simulink model "NetworkedControlSystemBasic_Part3"  (R2023b)
settings: Solver=FixedStepAuto  StartTime=0.0  StopTime=Tsim  FixedStep=Ts  RelTol=1e-3
values from neighbouring files (symbols this model uses):
  A = [0.9719 -0.0013;-0.0340 0.8628]    [Main_Part3.m]
  B = [-0.0839 0.0232;0.0761 0.4144]    [Main_Part3.m]
  C = [0 1]    [Main_Part3.m]
  D = [0 0]    [Main_Part3.m]
  K = lqi(sys,Q_LQI,R_LQ,0)    [Main_Part3.m]
  reference_time_vec = [0 100 250]    [Main_Part3.m]
  reference_value_vec = [0 10 17]    [Main_Part3.m]
  standardDeviationMeasurementNoise = 0.04    [Main_Part3.m]
  standardDeviationProcessNoise = 0.007    [Main_Part3.m]
  Ts = 1    [Main_Part3.m]
  x0 = zeros(size(A,1),1)    [Main_Part3.m]
  x0_hat = zeros(size(A,1),1)    [Main_Part3.m]
undefined symbols (not defined in the file or in its folder): DiscIntNeverNeededParam, L
settings Model: Creator=mehra  LastModifiedBy=amior
settings SolverCC: AlgebraicLoopSolver=TrustRegion
settings DebuggingCC: UnconnectedInputMsg=warning  UnconnectedOutputMsg=warning  UnconnectedLineMsg=warning
settings ModelReferenceCC: EnableRefExpFcnMdlSchedulingChecks=on
settings RTWCC: DLArmComputeVersion=19.05

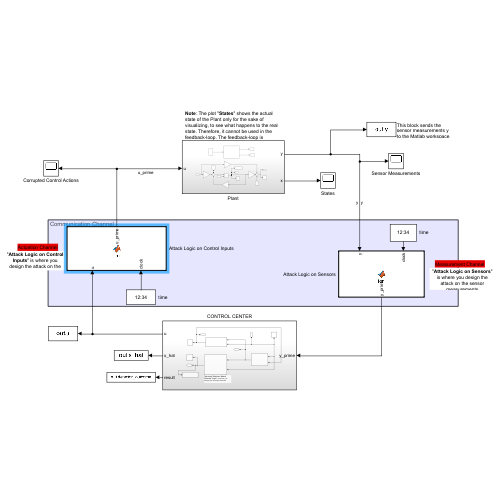
[thumbnail: Simulink's stored preview of the top-level diagram]
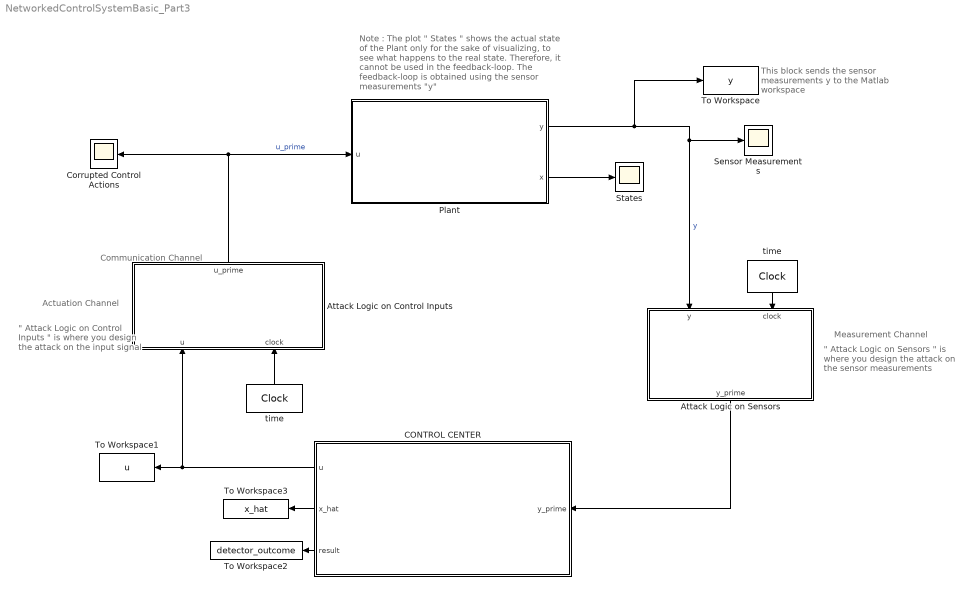
== system NetworkedControlSystemBasic_Part3 ==
  note: Note : The plot " States " shows the actual state of the Plant only for the sake of visualizing, to see what happens to the real state. Therefore, it cannot be used in the feedback-loop. The feedback-loop is obtained using the sensor measurements "y"
  note: Measurement Channel
  note: Actuation Channel
  note: Communication Channel
  note: " Attack Logic on Control Inputs " is where you design the attack on the input signal
  note: " Attack Logic on Sensors " is where you design the attack on the sensor measurements
  note: This block sends the sensor measurements y to the Matlab workspace
  Attack Logic on Control Inputs : MATLAB Function  TreatAsAtomicUnit=on
  Attack Logic on Sensors : MATLAB Function  TreatAsAtomicUnit=on
  CONTROL CENTER : Subsystem
  Corrupted Control Actions : Scope
  Plant : Subsystem
  "Sensor Measurements " : Scope
  States : Scope
  To Workspace : ToWorkspace  VariableName=y  SaveFormat=Structure With Time  SampleTime=Ts
  To Workspace1 : ToWorkspace  VariableName=u  SaveFormat=Structure With Time  SampleTime=Ts
  To Workspace2 : ToWorkspace  VariableName=detector_outcome  SaveFormat=Structure With Time  SampleTime=Ts
  To Workspace3 : ToWorkspace  VariableName=x_hat  SaveFormat=Structure With Time  SampleTime=Ts
  time : DigitalClock  SampleTime=Ts
  "time " : DigitalClock  SampleTime=Ts
  wires:
  "time "/1 -> Attack Logic on Sensors/2(clock)
  Attack Logic on Control Inputs/1(u_prime) -> Plant/1(u), Corrupted Control Actions/1  "u_prime"
  Plant/1(y) -> To Workspace/1, "Sensor Measurements "/1, Attack Logic on Sensors/1(y)  "y"
  time/1 -> Attack Logic on Control Inputs/2(clock)
  Plant/2(x) -> States/1
  CONTROL CENTER/1(u) -> Attack Logic on Control Inputs/1(u), To Workspace1/1
  Attack Logic on Sensors/1(y_prime) -> CONTROL CENTER/1(y_prime)
  CONTROL CENTER/2(x_hat) -> To Workspace3/1
  CONTROL CENTER/3(result) -> To Workspace2/1

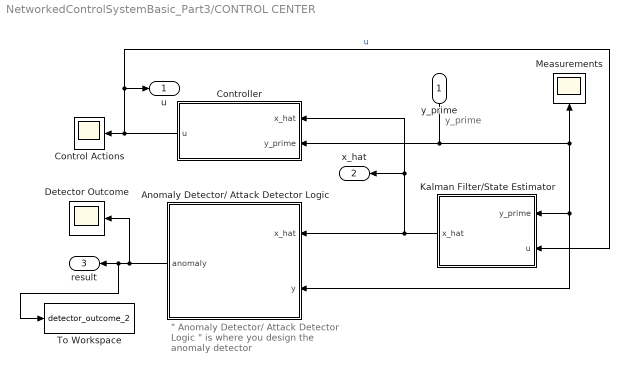
== system NetworkedControlSystemBasic_Part3/CONTROL CENTER ==
  note: y_prime
  note: " Anomaly Detector/ Attack Detector Logic " is where you design the anomaly detector
  y_prime : Inport
  Anomaly Detector/ Attack Detector Logic : MATLAB Function  TreatAsAtomicUnit=on
  Control Actions : Scope
  Controller : Subsystem
  Detector Outcome : Scope
  Kalman Filter/State Estimator : Subsystem
  Measurements : Scope
  To Workspace : ToWorkspace  VariableName=detector_outcome_2  SaveFormat=Structure With Time  SampleTime=-1
  u : Outport
  x_hat : Outport  Port=2
  result : Outport  Port=3
  wires:
  y_prime/1 -> Controller/2(y_prime), Kalman Filter/State Estimator/1(y_prime), Anomaly Detector/ Attack Detector Logic/2(y), Measurements/1
  Anomaly Detector/ Attack Detector Logic/1(anomaly) -> Detector Outcome/1, To Workspace/1, result/1
  Controller/1(u) -> u/1, Kalman Filter/State Estimator/2(u), Control Actions/1  "u"
  Kalman Filter/State Estimator/1(x_hat) -> Controller/1(x_hat), x_hat/1, Anomaly Detector/ Attack Detector Logic/1(x_hat)

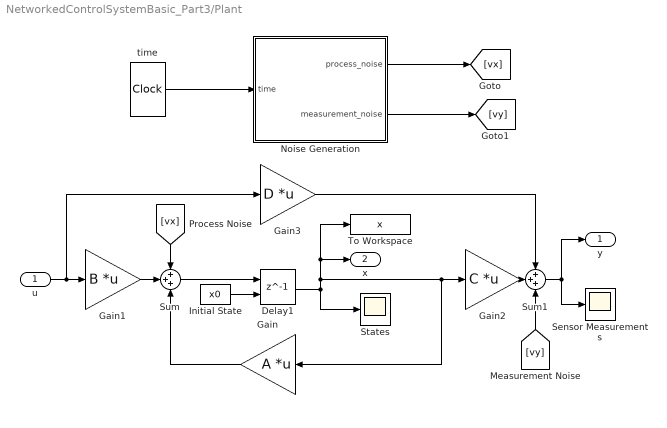
== system NetworkedControlSystemBasic_Part3/Plant ==
  u : Inport
  Delay1 : Delay  DelayLength=1  InitialConditionSource=Input port  InitialCondition=x0  SampleTime=Ts
      settings: InputPortMap=u0,p4
  Gain : Gain  Gain=A  Multiplication=Matrix(K*u)
  Gain1 : Gain  Gain=B  Multiplication=Matrix(K*u)
  Gain2 : Gain  Gain=C  Multiplication=Matrix(K*u)
  Gain3 : Gain  Gain=D  Multiplication=Matrix(K*u)
  Initial State : Constant  Value=x0
  Noise Generation : Subsystem
  Sensor Measurements : Scope
  States : Scope
  Sum : Sum  Inputs=+++
  Sum1 : Sum  Inputs=+++
  To Workspace : ToWorkspace  VariableName=x  SaveFormat=Structure With Time  SampleTime=Ts
  "time " : DigitalClock  SampleTime=Ts
  y : Outport  VectorParamsAs1DForOutWhenUnconnected=off
  x : Outport  Port=2  VectorParamsAs1DForOutWhenUnconnected=off
  wires:
  "time "/1 -> Noise Generation/1(time)
  Noise Generation/1(process_noise) -> [vx]
  Noise Generation/2(measurement_noise) -> [vy]
  Delay1/1 -> Gain2/1, Gain/1, x/1, To Workspace/1, States/1
  Sum/1 -> Delay1/1
  Gain/1 -> Sum/3
  Gain1/1 -> Sum/2
  u/1 -> Gain3/1, Gain1/1
  Gain2/1 -> Sum1/2
  Gain3/1 -> Sum1/1
  Sum1/1 -> Sensor Measurements/1, y/1
  [vx] -> Sum/1
  [vy] -> Sum1/3
  Initial State/1 -> Delay1/2

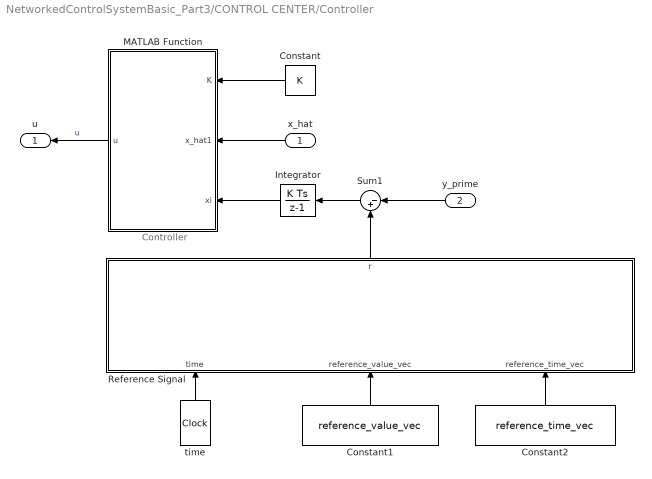
== system NetworkedControlSystemBasic_Part3/CONTROL CENTER/Controller ==
  note: Controller
  x_hat : Inport
  y_prime : Inport  Port=2
  Constant : Constant  Value=K  VectorParams1D=off
  Constant1 : Constant  Value=reference_value_vec  VectorParams1D=off
  Constant2 : Constant  Value=reference_time_vec  VectorParams1D=off
  Integrator : DiscreteIntegrator  SampleTime=Ts  ICPrevOutput=DiscIntNeverNeededParam  ICPrevScaledInput=DiscIntNeverNeededParam
  MATLAB Function : MATLAB Function  TreatAsAtomicUnit=on
  Reference Signal : MATLAB Function  TreatAsAtomicUnit=on
  Sum1 : Sum  Inputs=|-+
  "time   " : DigitalClock  SampleTime=Ts
  u : Outport  VectorParamsAs1DForOutWhenUnconnected=off
  wires:
  Sum1/1 -> Integrator/1
  x_hat/1 -> MATLAB Function/2(x_hat1)
  MATLAB Function/1(u) -> u/1  "u"
  y_prime/1 -> Sum1/1
  Integrator/1 -> MATLAB Function/3(xi)
  Reference Signal/1(r) -> Sum1/2
  "time   "/1 -> Reference Signal/1(time)
  Constant/1 -> MATLAB Function/1(K)
  Constant1/1 -> Reference Signal/2(reference_value_vec)
  Constant2/1 -> Reference Signal/3(reference_time_vec)

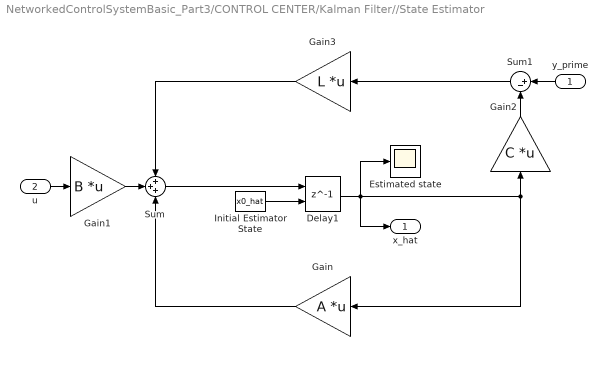
== system NetworkedControlSystemBasic_Part3/CONTROL CENTER/Kalman Filter//State Estimator ==
  y_prime : Inport
  u : Inport  Port=2
  Delay1 : Delay  DelayLength=1  InitialConditionSource=Input port  InitialCondition=x0  SampleTime=Ts
      settings: InputPortMap=u0,p4
  Estimated state : Scope
  Gain : Gain  Gain=A  Multiplication=Matrix(K*u)
  Gain1 : Gain  Gain=B  Multiplication=Matrix(K*u)
  Gain2 : Gain  Gain=C  Multiplication=Matrix(K*u)
  Gain3 : Gain  Gain=L  Multiplication=Matrix(K*u)
  Initial Estimator State : Constant  Value=x0_hat
  Sum : Sum  Inputs=+++
  Sum1 : Sum  Inputs=|+-
  x_hat : Outport  VectorParamsAs1DForOutWhenUnconnected=off
  wires:
  Gain3/1 -> Sum/1
  Initial Estimator State/1 -> Delay1/2
  Gain/1 -> Sum/3
  y_prime/1 -> Sum1/1
  Gain2/1 -> Sum1/2
  u/1 -> Gain1/1
  Sum1/1 -> Gain3/1
  Delay1/1 -> Gain/1, Gain2/1, Estimated state/1, x_hat/1
  Gain1/1 -> Sum/2
  Sum/1 -> Delay1/1

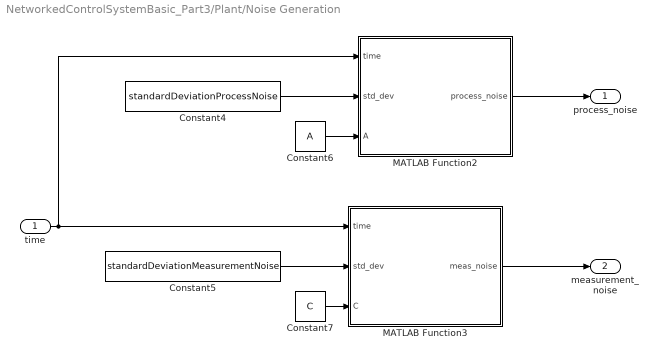
== system NetworkedControlSystemBasic_Part3/Plant/Noise Generation ==
  time : Inport
  Constant4 : Constant  Value=standardDeviationProcessNoise  VectorParams1D=off
  Constant5 : Constant  Value=standardDeviationMeasurementNoise  VectorParams1D=off
  Constant6 : Constant  Value=A  VectorParams1D=off
  Constant7 : Constant  Value=C  VectorParams1D=off
  MATLAB Function2 : MATLAB Function  TreatAsAtomicUnit=on
  MATLAB Function3 : MATLAB Function  TreatAsAtomicUnit=on
  process_noise : Outport
  measurement_noise : Outport  Port=2
  wires:
  Constant5/1 -> MATLAB Function3/2(std_dev)
  MATLAB Function3/1(meas_noise) -> measurement_noise/1
  time/1 -> MATLAB Function2/1(time), MATLAB Function3/1(time)
  Constant4/1 -> MATLAB Function2/2(std_dev)
  MATLAB Function2/1(process_noise) -> process_noise/1
  Constant7/1 -> MATLAB Function3/3(C)
  Constant6/1 -> MATLAB Function2/3(A)

== matlab function NetworkedControlSystemBasic_Part3/Attack Logic on Sensors ==
  data: y input; y_prime output; clock input
function y_prime = fcn(y, clock)

t = clock;

persistent y_history
if isempty(y_history)
    y_history = zeros(1, 401);
end

if t <= 400
    y_history(t + 1) = y;
end

if t < 240
    ya = 0;
elseif t <= 280
    ya = -y + y_history(t - 40 + 1);
else
    ya = 0;
end

y_prime = y + ya;
end

== matlab function NetworkedControlSystemBasic_Part3/CONTROL CENTER/Controller/MATLAB Function ==
  data: K input; x_hat1 input; u output; xi input
function u  = Controller(K,x_hat1,xi)
% This function contains controller's logic 
u=zeros(size(K,1),1);
x=[x_hat1;xi];

u=-K*x;

== matlab function NetworkedControlSystemBasic_Part3/Attack Logic on Control Inputs ==
  data: u input; u_prime output size=size(B,2); clock input
function u_prime = fcn(u, clock)

t = clock;

if t < 239
    ua = [0; 0];
elseif t < 280
    ua = -u + [0; 0.05 * (t - 240)];
else
    ua = [0; 0];
end

u_prime = u + ua;
end

== matlab function NetworkedControlSystemBasic_Part3/CONTROL CENTER/Anomaly Detector// Attack Detector Logic ==
  data: x_hat input; anomaly output; y input
function anomaly = Detector(x_hat, y)

% Output matrix
C = [0 1];

% Residual
r = y - C * x_hat;

% Residual covariance (scalar)
Sigma = 0.0016;

% Chi-squared test statistic
z = (r') * (1 / Sigma) * r;

% Threshold
alpha = 0.03;               % 3% false alarm rate
v = 1;                      % Residual is scalar
tau = chi2inv(1 - alpha, v);

% Detection decision
if z <= tau
    anomaly = 0;
else
    anomaly = 1;
end

% Log z(k) to base workspace for plotting
persistent z_log
if isempty(z_log)
    z_log = [];
end
z_log(end+1) = z;

assignin('base', 'z_log', z_log);
assignin('base', 'last_result', anomaly);
end

== matlab function NetworkedControlSystemBasic_Part3/CONTROL CENTER/Controller/Reference Signal ==
  data: r output; time input; reference_value_vec input; reference_time_vec input
function r = fcn(time,reference_value_vec,reference_time_vec)
%#codegen
% This function contains reference values 
search=true;
index=1;
r=zeros(size(reference_value_vec,1),1);



while search && size(reference_value_vec,2)>index
    if time>=reference_time_vec(index) && time<=reference_time_vec(index+1)
        search=false;
    else
        index=index+1;
    end
end
if index>size(reference_value_vec,2)
    index=size(reference_value_vec,2);
end


r=reference_value_vec(:,index);

== matlab function NetworkedControlSystemBasic_Part3/Plant/Noise Generation/MATLAB Function2 ==
  data: time input; process_noise output; std_dev input; A input
function process_noise = fcn(time,std_dev,A)

if time==0
    rng shuffle %this makes sure that everytime I run this simulink file, the noise is different
end

process_noise=normrnd(zeros(size(A,1),1),std_dev*ones(size(A,1),1));

return

== matlab function NetworkedControlSystemBasic_Part3/Plant/Noise Generation/MATLAB Function3 ==
  data: time input; meas_noise output; std_dev input; C input
function meas_noise = fcn(time,std_dev,C)

if time==0
    rng shuffle  %this makes sure that everytime I run this simulink file, the noise is different
end

meas_noise=normrnd(zeros(size(C,1),1),std_dev*ones(size(C,1),1));

return
